simulink model "lab_5_qpsk_pass_viterbi_sqrt_equalizer"  (R2012b)
settings: Solver=ode45  SolverMode=SingleTasking  StartTime=0.0  StopTime=0.0313  RelTol=1e-3
values from neighbouring files (symbols this model uses):
  EbNodB = EbNoVec(n)    [a1.m]    (also in a2.m = 11; cawgn.m = (1/4) * Nvar + 5; lab_5_Pber.m = 13; lab_5_Propyskna_Zdatnist.m = 11)
  Fc = 2*pi*Rs    (= 43.9822971503)    [lab_5_parameters.m]
  Rb = Nvar    (= 24)    [lab_5_Propyskna_Zdatnist.m]    (also in lab_5_parameters.m = 14)
  Tb = 1/Rb    (= 0.0416666666667)    [lab_5_Propyskna_Zdatnist.m]    (also in lab_5_parameters.m = 0.0714285714286)
  Td = Ts/128    (= 0.00111607142857)    [lab_5_parameters.m]
  Ts = 1/Rs    (= 0.142857142857)    [lab_5_parameters.m]
undefined symbols (not defined in the file or in its folder): dfilt, figposition, Fs, pskmod
libraries: commsink2 x8, dsparch4 x5, dspsrcs4 x4, commfilt2 x4, dspsnks4 x4, commchan3 x3, dspsigops x2, commcnvcod2 x2, dspobslib x2, commdigbbndpm3 x2, commrandsrc2 x1, dspindex x1
CloseFcn:
  | clear convSigsOut
settings Model: RequirementInfo=9  CovMetricSettings=d  ExtModeTrigMode=oneshot  ExtModeArmWhenConnect=off  Creator=mikem  LastModifiedBy=yuw
settings DataIOCC: LimitDataPoints=off  SaveOutput=off  SaveTime=off  SignalLoggingName=convSigsOut
settings OptimizationCC: BlockReduction=off  BooleanDataType=off  InitFltsAndDblsToZero=on
settings DebuggingCC: SaveWithParameterizedLinksMsg=none  SignalResolutionControl=TryResolveAllWithWarning  SolverPrmCheckMsg=none  MultiTaskDSMMsg=warning  MultiTaskCondExecSysMsg=none  IntegerOverflowMsg=none  StrictBusMsg=None
settings HardwareCC: TargetUnknown=on
settings RTWCC: IncludeERTFirstTime=on
settings GRTTargetCC: TargetFcnLib=ansi_tfl_tmw.mat  CombineOutputUpdateFcns=off  GRTInterface=on

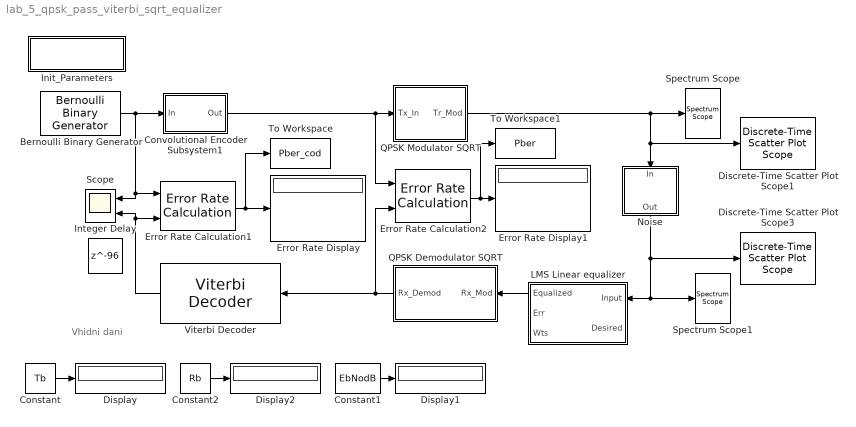
== system lab_5_qpsk_pass_viterbi_sqrt_equalizer ==
  note: Vhidni dani
  Bernoulli Binary Generator : commrandsrc2/Bernoulli Binary Generator  P=0.5  seed=12345  Ts=Tb  frameBased=on  sampPerFrame=1  orient=off  outDataType=double
  Constant : Constant  Value=Tb
  Constant1 : Constant  Value=EbNodB
  Constant2 : Constant  Value=Rb
  Convolutional Encoder Subsystem1 : Subsystem
  Discrete-Time Scatter Plot Scope1 : commsink2/Discrete-Time Scatter Plot Scope  Tag=ScatterPlot  sampPerSymb=1  offsetEye=0  numTraces=40  numNewFrames=10  LineMarkers=.  LineColors=b  fading=on  render=on  AxisGrid=on  xMin=-1.5  xMax=1.5  yMin=-1.5  yMax=1.5  inphaseLabel=In-phase Amplitude  quadratureLabel=Quadrature Amplitude  openScopeAtSimStart=off  FrameNumber=off  FigPos=[360 138 560 560]  figTitle=Scatter Plot  numLinesMax=8  block_type_=scatter
  Discrete-Time Scatter Plot Scope3 : commsink2/Discrete-Time Scatter Plot Scope  Tag=ScatterPlot  sampPerSymb=1  offsetEye=0  numTraces=40  numNewFrames=10  LineMarkers=.  LineColors=b  fading=on  render=on  AxisGrid=on  xMin=-1.5  xMax=1.5  yMin=-1.5  yMax=1.5  inphaseLabel=In-phase Amplitude  quadratureLabel=Quadrature Amplitude  openScopeAtSimStart=off  FrameNumber=off  FigPos=[360 138 560 560]  figTitle=Scatter Plot  numLinesMax=8  block_type_=scatter
  Display : Display
  Display1 : Display
  Display2 : Display
  Error Rate Calculation1 : commsink2/Error Rate Calculation  N=96  st_delay=0  cp_mode=Entire frame  subframe=[]  PMode=Port  WsName=ErrorVec  RsMode2=off  stop=off  numErr=100  maxBits=1e7
  Error Rate Calculation2 : commsink2/Error Rate Calculation  N=0  st_delay=0  cp_mode=Entire frame  subframe=[]  PMode=Port  WsName=ErrorVec  RsMode2=off  stop=off  numErr=100  maxBits=1e6
  Error Rate Display : Display
  Error Rate Display1 : Display
  Init_Parameters : Subsystem
      settings: OpenFcn=lab_5_parameters
      mask Display: disp('lab_5_parameters')
  Integer Delay : Delay  DelayLength=96  InputProcessing=Inherited
  LMS Linear equalizer : Subsystem
  Noise : Subsystem
  QPSK Demodulator SQRT : Subsystem
  QPSK Modulator SQRT : Subsystem
  Scope : Scope  NumInputPorts=2
      settings: YMin=-2~-2  YMax=2~2
  Spectrum Scope : dspsnks4/Spectrum Scope  ScopeProperties=on  Domain=Frequency  HorizSpan=1  UseBuffer=on  BufferSize=256  Overlap=0  TreatMby1Signals=M channels  inpFftLenInherit=off  FFTlength=128  numAvg=20  DisplayProperties=off  AxisGrid=on  Memory=off  FrameNumber=off  AxisLegend=off  AxisZoom=off  OpenScopeAtSimStart=off  OpenScopeImmediately=off  FigPos="figposition([7    12    39    27])"  AxisProperties=off  XUnits=Hertz  XRange=[-Fs/2...Fs/2]  XDisplay=0  InheritXIncr=on  XIncr=1.0  XLabel=Samples  XLimit=Auto  YUnits=dBW/Hertz  XMax=1  XMin=0  YLabel=Magnitude-squared, dB  LineProperties=off  LineColors=[1 0 0]  wintypeSpecScope=Hann  RsSpecScope=50  betaSpecScope=5  winsampSpecScope=Periodic  XAxisParamsVer=6.8  isFrameUpgraded=on
      settings: YMin=-50  YMax=10
  Spectrum Scope1 : dspsnks4/Spectrum Scope  ScopeProperties=on  Domain=Frequency  HorizSpan=1  UseBuffer=on  BufferSize=256  Overlap=0  TreatMby1Signals=M channels  inpFftLenInherit=off  FFTlength=128  numAvg=20  DisplayProperties=off  AxisGrid=on  Memory=off  FrameNumber=off  AxisLegend=off  AxisZoom=off  OpenScopeAtSimStart=off  OpenScopeImmediately=off  FigPos="figposition([49    12    39    27])"  AxisProperties=off  XUnits=Hertz  XRange=[-Fs/2...Fs/2]  XDisplay=0  InheritXIncr=on  XIncr=1.0  XLabel=Samples  XLimit=Auto  YUnits=dB  XMax=1  XMin=0  YLabel=Magnitude-squared, dB  LineProperties=off  LineColors=[1 0 0]  wintypeSpecScope=Hann  RsSpecScope=50  betaSpecScope=5  winsampSpecScope=Periodic  XAxisParamsVer=6.8  isFrameUpgraded=on
      settings: YMin=-10  YMax=10
  To Workspace : ToWorkspace  VariableName=Pber_cod  SampleTime=-1
      settings: MaxDataPoints=1
  To Workspace1 : ToWorkspace  VariableName=Pber  SampleTime=-1
      settings: MaxDataPoints=1
  Viterbi Decoder : commcnvcod2/Viterbi Decoder  trellis=poly2trellis(7, [171 133])  isPunctured=off  punctureVector=[1; 1; 0; 1; 0; 1]  erasures=off  dectype=Hard decision  runSigValErrCheck=off  nsdecb=4  smWordLength=16  tbdepth=96  opmode=Continuous  reset=off  outDataType=double  delayedResetAction=off
  wires:
  Error Rate Calculation1/1 -> To Workspace/1, Error Rate Display/1
  Convolutional Encoder Subsystem1/1(Out) -> Error Rate Calculation2/1, QPSK Modulator SQRT/1(Tx_In)
  Bernoulli Binary Generator/1 -> Error Rate Calculation1/1, Scope/1, Convolutional Encoder Subsystem1/1(In)
  Constant/1 -> Display/1
  Constant1/1 -> Display1/1
  Constant2/1 -> Display2/1
  Error Rate Calculation2/1 -> Error Rate Display1/1, To Workspace1/1
  Viterbi Decoder/1 -> Scope/2, Error Rate Calculation1/2
  QPSK Modulator SQRT/1(Tr_Mod) -> Spectrum Scope/1, Noise/1(In), Discrete-Time Scatter Plot Scope1/1
  Noise/1(Out) -> LMS Linear equalizer/1(Input), Spectrum Scope1/1, Discrete-Time Scatter Plot Scope3/1
  QPSK Demodulator SQRT/1(Rx_Demod) -> Viterbi Decoder/1, Error Rate Calculation2/2
  LMS Linear equalizer/1(Equalized) -> QPSK Demodulator SQRT/1(Rx_Mod)

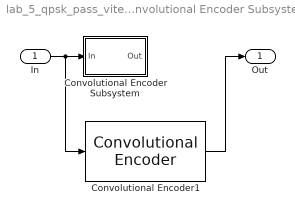
== system lab_5_qpsk_pass_viterbi_sqrt_equalizer/Convolutional Encoder Subsystem1 ==
  In : Inport
  Convolutional Encoder Subsystem : Subsystem
  Convolutional Encoder1 : commcnvcod2/Convolutional Encoder  trellis=poly2trellis(7, [171 133])  opMode=Continuous  DelayedResetAction=off  hasIniStPort=off  hasFinStPort=off  usePuncVector=off  punctureVector=[1; 1; 0; 1; 0; 1]  reset=Unused parameter value
  Out : Outport
  wires:
  In/1 -> Convolutional Encoder Subsystem/1(In), Convolutional Encoder1/1
  Convolutional Encoder1/1 -> Out/1

== system lab_5_qpsk_pass_viterbi_sqrt_equalizer/Init_Parameters ==

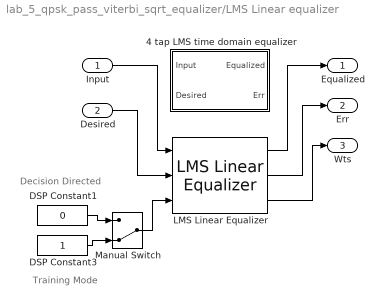
== system lab_5_qpsk_pass_viterbi_sqrt_equalizer/LMS Linear equalizer ==
  note: Decision Directed
  note: Training Mode
  Input : Inport
  Desired : Inport  Port=2
  4 tap LMS time domain equalizer : Subsystem
  DSP Constant1 : Constant  Value=0  VectorParams1D=off  FramePeriod=1
      settings: SamplingMode=Frame based
  DSP Constant3 : Constant  VectorParams1D=off  FramePeriod=1
      settings: SamplingMode=Frame based
  LMS Linear Equalizer : commeq2/LMS Linear  Equalizer  nTaps=4  nSamp=1  sigConst=pskmod([0:4-1],4)  delay=2  stepSize=0.01  leakage=1  initWeights=0  mode=on  outErr=on  outWeights=on
  Manual Switch : ManualSwitch  CurrentSetting=0
  Equalized : Outport
  Err : Outport  Port=2
  Wts : Outport  Port=3
  wires:
  Input/1 -> LMS Linear Equalizer/1
  Desired/1 -> LMS Linear Equalizer/2
  LMS Linear Equalizer/3 -> Wts/1
  LMS Linear Equalizer/2 -> Err/1
  LMS Linear Equalizer/1 -> Equalized/1
  Manual Switch/1 -> LMS Linear Equalizer/3
  DSP Constant3/1 -> Manual Switch/2
  DSP Constant1/1 -> Manual Switch/1

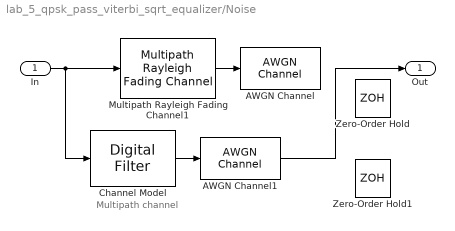
== system lab_5_qpsk_pass_viterbi_sqrt_equalizer/Noise ==
  note: Multipath channel
  In : Inport
  AWGN Channel : commchan3/AWGN Channel  InputProcessing=Inherited (this choice will be removed - see release notes)  seed=67  noiseMode="Signal to noise ratio  (Eb/No)"  EbNodB=10  EsNodB=10  SNRdB=10  bitsPerSym=1  Ps=1  Tsym=1  variance=1
  AWGN Channel1 : commchan3/AWGN Channel  InputProcessing=Inherited (this choice will be removed - see release notes)  seed=67  noiseMode="Signal to noise ratio  (SNR)"  EbNodB=10  EsNodB=10  SNRdB=40  bitsPerSym=1  Ps=1  Tsym=1  variance=1
  Channel Model : dsparch4/Digital Filter  TypePopup=FIR (all zeros)  IIRFiltStruct=Direct form I transposed  AllPoleFiltStruct=Direct form transposed  FIRFiltStruct=Direct form transposed  CoeffSource=Specify via dialog  NumCoeffs=[1 -.3 .1 .2j]  DenCoeffs=[1 0.1]  BiQuadCoeffs=[1 0.3 0.4 1 0.1 0.2]  LatticeCoeffs=[0.2 0.4]  denIgnore=on  FiltPerSampPopup=One filter per frame  IC=0  ICnum=0  ICden=0  roundingMode=Floor  overflowMode=off  ScaleValues=1  scaleValueFracLength=14  stageInFracLength=15  stageOutFracLength=15  FilterSource=Specify via dialog  dfiltObjectName=dfilt.dffir([1 2 1])  InputProcessing=Inherited (this choice will be removed - see release notes)
  Multipath Rayleigh Fading Channel1 : commchan3/Multipath Rayleigh Fading Channel  maxDopplerShift=40  spectrumType=Jakes  sigmaGaussian=1/sqrt(2)  coeffRounded=[1 -1.72 0.785]  freqMinMaxRJakes=[0 1]  freqMinMaxAJakes=[0 1]  sigmaGaussian1=1/sqrt(2)  sigmaGaussian2=1/sqrt(2)  centerFreqGaussian1=0.0  centerFreqGaussian2=0.0  gainGaussian1=0.5  gainGaussian2=0.5  coeffBell=9  dopplerSpectrum=doppler.jakes  pathDelays=[0 2e-6]  avgPathGaindB=[0 -3]  normalizePathGains=on  seed=73  enableProbe=0  openVisAtStart=off  outPathGains=off  outDelay=off
  Zero-Order Hold : ZeroOrderHold  SampleTime=Td
  Zero-Order Hold1 : ZeroOrderHold  SampleTime=Td
  Out : Outport
  wires:
  In/1 -> Multipath Rayleigh Fading Channel1/1, Channel Model/1
  AWGN Channel1/1 -> Out/1
  Channel Model/1 -> AWGN Channel1/1
  Multipath Rayleigh Fading Channel1/1 -> AWGN Channel/1

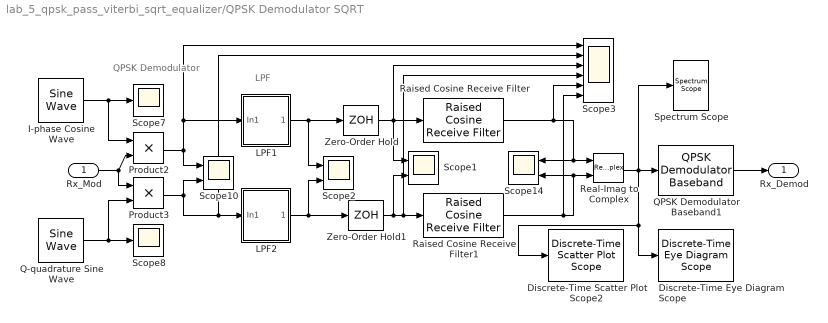
== system lab_5_qpsk_pass_viterbi_sqrt_equalizer/QPSK Demodulator SQRT ==
  note: LPF
  note: QPSK Demodulator
  Rx_Mod : Inport
  Discrete-Time Eye Diagram Scope : commsink2/Discrete-Time Eye Diagram Scope  Tag=EyeDiagram  sampPerSymb=8  offsetEye=0  symbPerTrace=1  numTraces=40  numNewFrames=10  LineStyles=-  LineColors=b  dupPoints=on  fading=on  render=on  AxisGrid=on  yMin=-1.5  yMax=1.5  inphaseLabel=In-phase Amplitude  quadratureLabel=Quadrature Amplitude  openScopeAtSimStart=off  dispDiagram=In-phase and Quadrature  FrameNumber=off  FigPos=[360 54 560 644]  figTitle=Eye Diagram  block_type_=eye  numLinesMax=8
  Discrete-Time Scatter Plot Scope2 : commsink2/Discrete-Time Scatter Plot Scope  Tag=ScatterPlot  sampPerSymb=1  offsetEye=0  numTraces=40  numNewFrames=10  LineMarkers=.  LineColors=b  fading=on  render=on  AxisGrid=on  xMin=-1.5  xMax=1.5  yMin=-1.5  yMax=1.5  inphaseLabel=In-phase Amplitude  quadratureLabel=Quadrature Amplitude  openScopeAtSimStart=off  FrameNumber=off  FigPos=[360 138 560 560]  figTitle=Scatter Plot  numLinesMax=8  block_type_=scatter
  I-phase Cosine Wave : dspsrcs4/Sine Wave  Amplitude=sqrt(2)  Frequency=Fc  Phase=pi/2  SampleMode=Discrete  OutComplex=Real  CompMethod=Trigonometric fcn  TableSize=Speed  SampleTime=Td  SamplesPerFrame=1  ResetState=Restart at time zero  dataType=double  wordLen=16  udDataType=sfix(16)  fracBitsMode=Best precision  numFracBits=15  OutDataTypeStr=double  LastOutDataTypeStr=double
  LPF1 : Subsystem
  LPF2 : Subsystem
  Product2 : Product  SampleTime=Td  RndMeth=Zero
  Product3 : Product  SampleTime=Td  RndMeth=Zero
  Q-quadrature Sine Wave : dspsrcs4/Sine Wave  Amplitude=1  Frequency=Fc  Phase=pi  SampleMode=Discrete  OutComplex=Real  CompMethod=Trigonometric fcn  TableSize=Speed  SampleTime=Td  SamplesPerFrame=1  ResetState=Restart at time zero  dataType=double  wordLen=16  udDataType=sfix(16)  fracBitsMode=Best precision  numFracBits=15  OutDataTypeStr=double  LastOutDataTypeStr=double
  QPSK Demodulator Baseband1 : commdigbbndpm3/QPSK Demodulator Baseband  Ph=pi/4  Dec=Gray  OutType=Integer  DecType=Hard decision  VarSource=Dialog  Variance=1  outDtype1=Inherit via internal rule  outDtype2=Inherit via internal rule  derotateFactorWordLen=16
  Raised Cosine Receive Filter : commfilt2/Raised Cosine Receive Filter  filtType=Square root  N=8  D=6  R=0.2  sampMode=Mute  saveAsFlag=0  rateMode=Downsampling  downFactor=8  downOffset=0  framing=Maintain input frame size  InputProcessing=Inherited (this choice will be removed - see release notes)  checkGain=Normalized  filterGain=1  checkCoeff=off  variableName=rcRxFilt  launchFVT=off  roundingMode=Floor  overflowMode=off
  Raised Cosine Receive Filter1 : commfilt2/Raised Cosine Receive Filter  filtType=Square root  N=8  D=6  R=0.2  sampMode=Mute  saveAsFlag=0  rateMode=Downsampling  downFactor=8  downOffset=0  framing=Maintain input frame size  InputProcessing=Inherited (this choice will be removed - see release notes)  checkGain=Normalized  filterGain=1  checkCoeff=off  variableName=rcRxFilt1  launchFVT=off  roundingMode=Floor  overflowMode=off
  Real-Imag to Complex : RealImagToComplex
  Scope{1..2,10,14} (4 alike) : Scope  NumInputPorts=2
      Scope1 settings: YMin=-5~-5  YMax=5~5  SaveName=ScopeData12
      Scope10 settings: YMin=-5~-5  YMax=5~5  SaveName=ScopeData10
      Scope14 settings: TimeRange=5  YMin=-5~-5  YMax=5~5  SaveName=ScopeData4
      Scope2 settings: YMin=-5~-5  YMax=5~5  SaveName=ScopeData14
  Scope3 : Scope  NumInputPorts=6
      settings: YMin=-5~-5~-5~-5~-5~-5  YMax=5~5~5~5~5~5  SaveName=ScopeData15
  Scope7 : Scope
      settings: SaveName=ScopeData7
  Scope8 : Scope
      settings: SaveName=ScopeData8
  Spectrum Scope : dspsnks4/Spectrum Scope  ScopeProperties=on  Domain=Frequency  HorizSpan=1  UseBuffer=on  BufferSize=256  Overlap=0  TreatMby1Signals=M channels  inpFftLenInherit=off  FFTlength=128  numAvg=20  DisplayProperties=off  AxisGrid=on  Memory=off  FrameNumber=off  AxisLegend=off  AxisZoom=off  OpenScopeAtSimStart=off  OpenScopeImmediately=off  FigPos="figposition([49    12    39    27])"  AxisProperties=off  XUnits=Hertz  XRange=[-Fs/2...Fs/2]  XDisplay=0  InheritXIncr=on  XIncr=1.0  XLabel=Samples  XLimit=Auto  YUnits=dB  XMax=1  XMin=0  YLabel=Magnitude-squared, dB  LineProperties=off  LineColors=[1 0 0]  wintypeSpecScope=Hann  RsSpecScope=50  betaSpecScope=5  winsampSpecScope=Periodic  XAxisParamsVer=6.8  isFrameUpgraded=on
      settings: YMin=-10  YMax=10
  Zero-Order Hold : ZeroOrderHold  SampleTime=Ts/8
  Zero-Order Hold1 : ZeroOrderHold  SampleTime=1/Rs/8
  Rx_Demod : Outport
  wires:
  Raised Cosine Receive Filter/1 -> Scope3/5, Scope14/1, Real-Imag to Complex/1
  Raised Cosine Receive Filter1/1 -> Scope3/6, Scope14/2, Real-Imag to Complex/2
  LPF2/1(Out1) -> Scope2/2, Zero-Order Hold1/1
  LPF1/1(Out1) -> Scope2/1, Zero-Order Hold/1
  Zero-Order Hold1/1 -> Scope3/4, Raised Cosine Receive Filter1/1, Scope1/2
  Zero-Order Hold/1 -> Scope3/3, Scope1/1, Raised Cosine Receive Filter/1
  QPSK Demodulator Baseband1/1 -> Rx_Demod/1
  Rx_Mod/1 -> Product3/1, Product2/2
  Q-quadrature Sine Wave/1 -> Product3/2, Scope8/1
  I-phase Cosine Wave/1 -> Product2/1, Scope7/1
  Product2/1 -> Scope3/1, LPF1/1(In1), Scope10/1
  Product3/1 -> Scope3/2, LPF2/1(In1), Scope10/2
  Real-Imag to Complex/1 -> QPSK Demodulator Baseband1/1, Spectrum Scope/1, Discrete-Time Scatter Plot Scope2/1, Discrete-Time Eye Diagram Scope/1

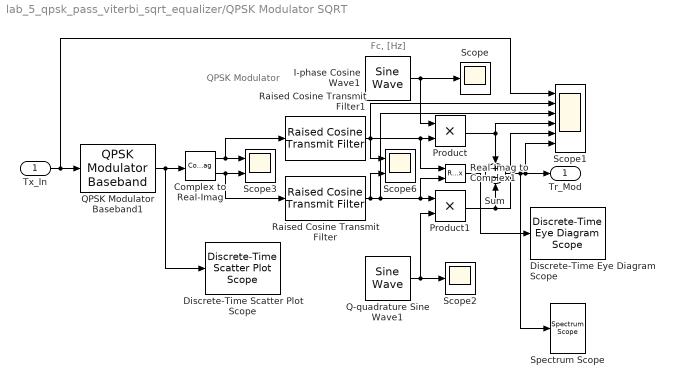
== system lab_5_qpsk_pass_viterbi_sqrt_equalizer/QPSK Modulator SQRT ==
  note: Fc, [Hz]
  note: QPSK Modulator
  Tx_In : Inport
  Complex to Real-Imag : ComplexToRealImag
  Discrete-Time Eye Diagram Scope : commsink2/Discrete-Time Eye Diagram Scope  Tag=EyeDiagram  sampPerSymb=8  offsetEye=0  symbPerTrace=1  numTraces=40  numNewFrames=10  LineStyles=-  LineColors=b  dupPoints=on  fading=on  render=on  AxisGrid=on  yMin=-1.5  yMax=1.5  inphaseLabel=In-phase Amplitude  quadratureLabel=Quadrature Amplitude  openScopeAtSimStart=off  dispDiagram=In-phase and Quadrature  FrameNumber=off  FigPos=[360 54 560 644]  figTitle=Eye Diagram  block_type_=eye  numLinesMax=8
  Discrete-Time Scatter Plot Scope : commsink2/Discrete-Time Scatter Plot Scope  Tag=ScatterPlot  sampPerSymb=1  offsetEye=0  numTraces=40  numNewFrames=10  LineMarkers=.  LineColors=b  fading=on  render=on  AxisGrid=on  xMin=-1.5  xMax=1.5  yMin=-1.5  yMax=1.5  inphaseLabel=In-phase Amplitude  quadratureLabel=Quadrature Amplitude  openScopeAtSimStart=off  FrameNumber=off  FigPos=[360 138 560 560]  figTitle=Scatter Plot  numLinesMax=8  block_type_=scatter
  I-phase Cosine Wave1 : dspsrcs4/Sine Wave  Amplitude=sqrt(2)  Frequency=Fc  Phase=pi/2  SampleMode=Discrete  OutComplex=Real  CompMethod=Trigonometric fcn  TableSize=Speed  SampleTime=Td  SamplesPerFrame=1  ResetState=Restart at time zero  dataType=double  wordLen=16  udDataType=sfix(16)  fracBitsMode=Best precision  numFracBits=15  OutDataTypeStr=double  LastOutDataTypeStr=double
  Product : Product  RndMeth=Zero
  Product1 : Product  RndMeth=Zero
  Q-quadrature Sine Wave1 : dspsrcs4/Sine Wave  Amplitude=1  Frequency=Fc  Phase=0  SampleMode=Discrete  OutComplex=Real  CompMethod=Trigonometric fcn  TableSize=Speed  SampleTime=Td  SamplesPerFrame=1  ResetState=Restart at time zero  dataType=double  wordLen=16  udDataType=sfix(16)  fracBitsMode=Best precision  numFracBits=15  OutDataTypeStr=double  LastOutDataTypeStr=double
  QPSK Modulator Baseband1 : commdigbbndpm3/QPSK Modulator Baseband  InType=Integer  Enc=Gray  Ph=pi/4  outDtype=double  outWordLen=16  outUDDataType=sfix(16)  outFracLenMode=Best precision  outFracLen=15
  Raised Cosine Transmit Filter : commfilt2/Raised Cosine Transmit Filter  filtType=Square root  D=6  R=0.2  sampMode=Mute  saveAsFlag=0  N=8  framing=Maintain input frame size  InputProcessing=Inherited (this choice will be removed - see release notes)  checkGain=Normalized  filterGain=1  checkCoeff=off  variableName=rcTxFilt  launchFVT=off  roundingMode=Floor  overflowMode=off
  Raised Cosine Transmit Filter1 : commfilt2/Raised Cosine Transmit Filter  filtType=Square root  D=6  R=0.2  sampMode=Mute  saveAsFlag=0  N=8  framing=Maintain input frame size  InputProcessing=Inherited (this choice will be removed - see release notes)  checkGain=Normalized  filterGain=1  checkCoeff=off  variableName=rcTxFilt1  launchFVT=off  roundingMode=Floor  overflowMode=off
  Real-Imag to Complex1 : RealImagToComplex
  Scope : Scope
      settings: SaveName=ScopeData2
  Scope1 : Scope  NumInputPorts=6
      settings: TimeRange=5  YMin=-5~-5~-5~-5~-5~-5  YMax=5~5~5~5~5~5
  Scope2 : Scope
      settings: SaveName=ScopeData3
  Scope3 : Scope  NumInputPorts=2
      settings: YMin=-5~-5  YMax=5~5  SaveName=ScopeData13
  Scope6 : Scope  NumInputPorts=2
      settings: YMin=-5~-5  YMax=5~5  SaveName=ScopeData6
  Spectrum Scope : dspsnks4/Spectrum Scope  ScopeProperties=on  Domain=Frequency  HorizSpan=1  UseBuffer=on  BufferSize=256  Overlap=0  TreatMby1Signals=M channels  inpFftLenInherit=off  FFTlength=128  numAvg=20  DisplayProperties=off  AxisGrid=on  Memory=off  FrameNumber=off  AxisLegend=off  AxisZoom=off  OpenScopeAtSimStart=off  OpenScopeImmediately=off  FigPos="figposition([49    12    39    27])"  AxisProperties=off  XUnits=Hertz  XRange=[-Fs/2...Fs/2]  XDisplay=0  InheritXIncr=on  XIncr=1.0  XLabel=Samples  XLimit=Auto  YUnits=dB  XMax=1  XMin=0  YLabel=Magnitude-squared, dB  LineProperties=off  LineColors=[1 0 0]  wintypeSpecScope=Hann  RsSpecScope=50  betaSpecScope=5  winsampSpecScope=Periodic  XAxisParamsVer=6.8  isFrameUpgraded=on
      settings: YMin=-10  YMax=10
  Sum : Sum  Inputs=+-
  Tr_Mod : Outport
  wires:
  Real-Imag to Complex1/1 -> Discrete-Time Eye Diagram Scope/1
  Complex to Real-Imag/2 -> Scope3/2, Raised Cosine Transmit Filter/1
  Complex to Real-Imag/1 -> Scope3/1, Raised Cosine Transmit Filter1/1
  Raised Cosine Transmit Filter1/1 -> Scope1/2, Real-Imag to Complex1/1, Product/2, Scope6/1
  Q-quadrature Sine Wave1/1 -> Scope2/1, Product1/2
  I-phase Cosine Wave1/1 -> Scope/1, Product/1
  Raised Cosine Transmit Filter/1 -> Scope1/3, Real-Imag to Complex1/2, Product1/1, Scope6/2
  Tx_In/1 -> QPSK Modulator Baseband1/1, Scope1/1
  Sum/1 -> Spectrum Scope/1, Scope1/6, Tr_Mod/1
  Product/1 -> Scope1/4, Sum/1
  QPSK Modulator Baseband1/1 -> Complex to Real-Imag/1, Discrete-Time Scatter Plot Scope/1
  Product1/1 -> Scope1/5, Sum/2

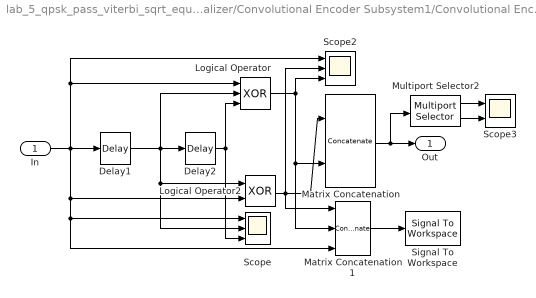
== system lab_5_qpsk_pass_viterbi_sqrt_equalizer/Convolutional Encoder Subsystem1/Convolutional Encoder Subsystem ==
  In : Inport
  Delay1 : dspsigops/Delay  InputProcessing=Inherited (this choice will be removed - see release notes)  dly_unit=Samples  delay=1  ic_detail=off  dif_ic_for_ch=off  dif_ic_for_dly=off  ic=0  reset_popup=None
  Delay2 : dspsigops/Delay  InputProcessing=Inherited (this choice will be removed - see release notes)  dly_unit=Samples  delay=1  ic_detail=off  dif_ic_for_ch=off  dif_ic_for_dly=off  ic=0  reset_popup=None
  Logical Operator : Logic  Operator=XOR  Inputs=3  AllPortsSameDT=off
  Logical Operator2 : Logic  Operator=XOR  AllPortsSameDT=off
  Matrix Concatenation : Concatenate  Mode=Multidimensional array
  Matrix Concatenation1 : Concatenate  NumInputs=3  Mode=Multidimensional array  ConcatenateDimension=2
  Multiport Selector2 : dspindex/Multiport Selector  rowsOrCols=Rows  idxCellArray={1 2}  idxErrMode=Clip Index
  Scope : Scope  NumInputPorts=3
      settings: YMin=-5~-5~-5  YMax=5~5~5
  Scope2 : Scope  NumInputPorts=3
      settings: YMin=-5~-5~-5  YMax=5~5~5  SaveName=ScopeData2
  Scope3 : Scope  NumInputPorts=2
      settings: YMin=-5~-5  YMax=5~5  SaveName=ScopeData3
  Signal To Workspace : SignalToWorkspace  VariableName=In_Cod
      settings: CopyFcn=dspblkcopystw(gcbh);
  Out : Outport
  wires:
  Delay2/1 -> Logical Operator/3, Scope/3
  Delay1/1 -> Delay2/1, Logical Operator/2, Scope/2, Logical Operator2/1
  Multiport Selector2/1 -> Scope3/1
  Multiport Selector2/2 -> Scope3/2
  Logical Operator/1 -> Scope2/3, Matrix Concatenation/2, Matrix Concatenation1/2
  Logical Operator2/1 -> Scope2/2, Matrix Concatenation/1, Matrix Concatenation1/1
  In/1 -> Delay1/1, Logical Operator2/2, Scope/1, Matrix Concatenation1/3, Logical Operator/1, Scope2/1
  Matrix Concatenation/1 -> Out/1, Multiport Selector2/1
  Matrix Concatenation1/1 -> Signal To Workspace/1

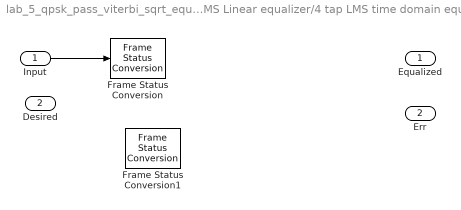
== system lab_5_qpsk_pass_viterbi_sqrt_equalizer/LMS Linear equalizer/4 tap LMS time domain equalizer ==
  Input : Inport
  Desired : Inport  Port=2
  Frame Status Conversion : dspobslib/Frame Status Conversion  growRefPort=off  outframe=Frame-based
  Frame Status Conversion1 : dspobslib/Frame Status Conversion  growRefPort=off  outframe=Frame-based
  Equalized : Outport
  Err : Outport  Port=2
  wires:
  Input/1 -> Frame Status Conversion/1

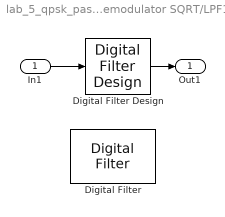
== system lab_5_qpsk_pass_viterbi_sqrt_equalizer/QPSK Demodulator SQRT/LPF1 ==
  In1 : Inport
  Digital Filter Design : dsparch4/Digital Filter Design  mwdsp_browser_bugfix_var=off
  Digital Filter : dsparch4/Digital Filter  TypePopup=FIR (all zeros)  IIRFiltStruct=Direct form II transposed  AllPoleFiltStruct=Direct form  FIRFiltStruct=Direct form  CoeffSource=Specify via dialog  NumCoeffs=[1 2]  DenCoeffs=[1 0.1]  BiQuadCoeffs=[1 0.3 0.4 1 0.1 0.2]  LatticeCoeffs=[0.2 0.4]  denIgnore=on  FiltPerSampPopup=One filter per frame  IC=0  ICnum=0  ICden=0  roundingMode=Floor  overflowMode=off  ScaleValues=1  scaleValueFracLength=14  stageInFracLength=15  stageOutFracLength=15  FilterSource=Specify via dialog  dfiltObjectName=dfilt.dffir([1 2 1])  InputProcessing=Inherited (this choice will be removed - see release notes)
  Out1 : Outport
  wires:
  In1/1 -> Digital Filter Design/1
  Digital Filter Design/1 -> Out1/1

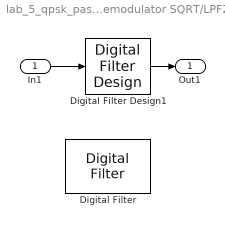
== system lab_5_qpsk_pass_viterbi_sqrt_equalizer/QPSK Demodulator SQRT/LPF2 ==
  In1 : Inport
  Digital Filter Design1 : dsparch4/Digital Filter Design  mwdsp_browser_bugfix_var=off
  Digital Filter : dsparch4/Digital Filter  TypePopup=IIR (poles & zeros)  IIRFiltStruct=Direct form II transposed  AllPoleFiltStruct=Direct form  FIRFiltStruct=Direct form  CoeffSource=Specify via dialog  NumCoeffs=[1 2]  DenCoeffs=[1 0.1]  BiQuadCoeffs=[1 0.3 0.4 1 0.1 0.2]  LatticeCoeffs=[0.2 0.4]  denIgnore=on  FiltPerSampPopup=One filter per frame  IC=0  ICnum=0  ICden=0  roundingMode=Floor  overflowMode=off  ScaleValues=1  scaleValueFracLength=14  stageInFracLength=15  stageOutFracLength=15  FilterSource=Specify via dialog  dfiltObjectName=dfilt.dffir([1 2 1])  InputProcessing=Inherited (this choice will be removed - see release notes)
  Out1 : Outport
  wires:
  In1/1 -> Digital Filter Design1/1
  Digital Filter Design1/1 -> Out1/1
